simulink model "PIDControllerPulse"  (R2025b)
settings: Solver=FixedStepAuto  StartTime=0.0  StopTime=inf  FixedStep=Ts  RelTol=1e-3
model workspace (MATLAB code in the model file):
  | motor_max_torque = 2.2;
  | gear_ratio = [70/16; 40/16; 1];
  | 
  | u_max =   motor_max_torque * gear_ratio;
  | u_min = - motor_max_torque * gear_ratio;
  | 
  | voltage_max    = 15;
  | torque2voltage = voltage_max ./ u_max;
  | 
  | Ts = 1e-3;
  | pp = 14;
undefined symbols (not defined in the file): effort, effort_SL_Info, position, position_SL_Info
libraries: ros2lib x3, slpidlib x1, eeGeneralControl x1
settings Model: Creator=Asus  LastModifiedBy=Asus
settings OptimizationCC: DefaultParameterBehavior=Inlined  EnhancedBackFolding=on  PassReuseOutputArgsAs=Individual arguments  ZeroExternalMemoryAtStartup=off  ZeroInternalMemoryAtStartup=off  MaxStackSize=64  OptimizeBlockOrder=speed  DifferentSizesBufferReuse=on  OptimizationCustomize=off  EfficientTunableParamExpr=on
settings DebuggingCC: ParameterTunabilityLossMsg=error
settings SFSimCC: MATLABDynamicMemAlloc=off
settings RTWCC: SystemTargetFile=ert.tlc  HardwareBoard=Robot Operating System 2 (ROS 2)  TLCOptions="-aInlineSetEventsForThisBaseRateFcn=TLC_FALSE -aSuppressMultiTaskScheduler=TLC_FALSE  -aRateBasedStepFcn=0"  TemplateMakefile=ert_default_tmf  Toolchain=Colcon Tools  TargetLang=C++  Description=Embedded Coder
settings CodeAppCC: ForceParamTrailComments=on  IgnoreCustomStorageClasses=off  MaxIdLength=95.0  OperatorAnnotations=on  SimulinkDataObjDesc=on  SFDataObjDesc=on  InsertBlockDesc=on
settings ERTTargetCC: RootIOFormat=Structure reference  CodeInterfacePackaging=C++ class

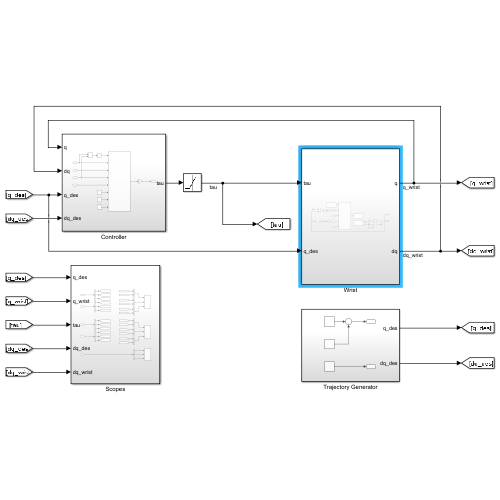
[thumbnail: Simulink's stored preview of the top-level diagram]
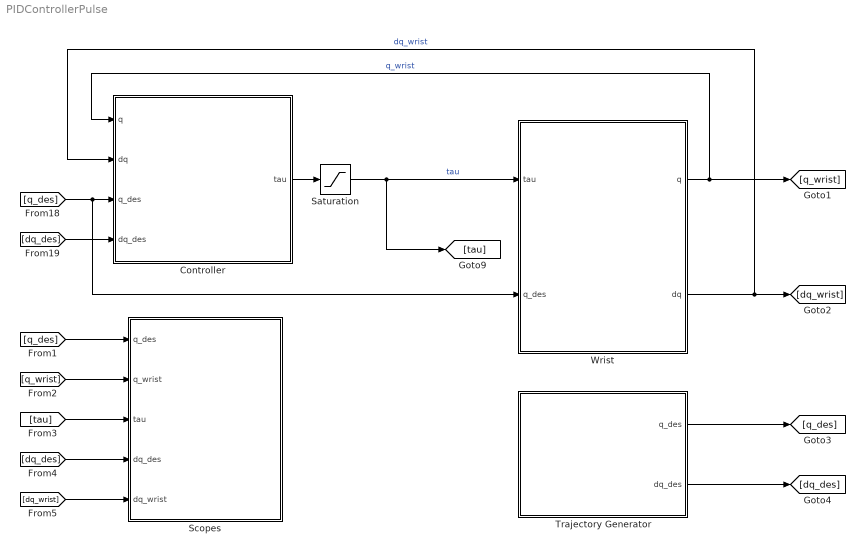
== system PIDControllerPulse ==
  Controller : Subsystem
  Saturation : Saturate  UpperLimit=u_max  LowerLimit=u_min
  Scopes : Subsystem
  Trajectory Generator : Subsystem
  Wrist : Subsystem
  wires:
  [q_des] -> Wrist/2(q_des), Controller/3(q_des)
  [dq_des] -> Controller/4(dq_des)
  Controller/1(tau) -> Saturation/1
  Wrist/1(q) -> Controller/1(q), [q_wrist]  "q_wrist"
  Wrist/2(dq) -> [dq_wrist], Controller/2(dq)  "dq_wrist"
  [q_des] -> Scopes/1(q_des)
  [q_wrist] -> Scopes/2(q_wrist)
  [tau] -> Scopes/3(tau)
  Trajectory Generator/1(q_des) -> [q_des]
  Trajectory Generator/2(dq_des) -> [dq_des]
  [dq_des] -> Scopes/4(dq_des)
  [dq_wrist] -> Scopes/5(dq_wrist)
  Saturation/1 -> [tau], Wrist/1(tau)  "tau"

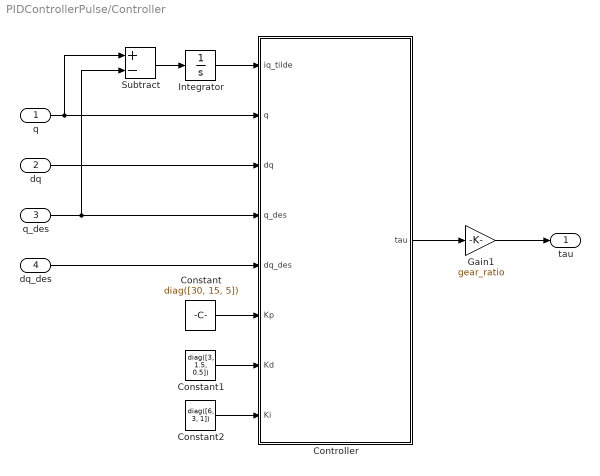
== system PIDControllerPulse/Controller ==
  q : Inport
  dq : Inport  Port=2
  q_des : Inport  Port=3
  dq_des : Inport  Port=4
  Constant : Constant  Value=diag([30, 15, 5])
  Constant1 : Constant  Value=diag([3, 1.5, 0.5])
  Constant2 : Constant  Value=diag([6, 3, 1])
  Controller : MATLAB Function  TreatAsAtomicUnit=on
  Gain1 : Gain  Gain=gear_ratio
  Integrator : Integrator  InitialCondition=zeros(3, 1)
  Subtract : Sum  Inputs=+-
  tau : Outport
  wires:
  q_des/1 -> Subtract/2, Controller/4(q_des)
  dq/1 -> Controller/3(dq)
  q/1 -> Subtract/1, Controller/2(q)
  Constant/1 -> Controller/6(Kp)
  Constant1/1 -> Controller/7(Kd)
  dq_des/1 -> Controller/5(dq_des)
  Subtract/1 -> Integrator/1
  Integrator/1 -> Controller/1(iq_tilde)
  Constant2/1 -> Controller/8(Ki)
  Controller/1(tau) -> Gain1/1
  Gain1/1 -> tau/1

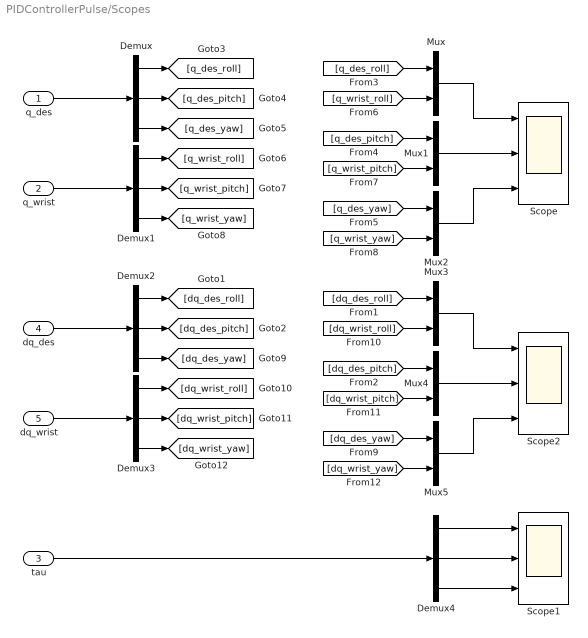
== system PIDControllerPulse/Scopes ==
  q_des : Inport
  q_wrist : Inport  Port=2
  tau : Inport  Port=3
  dq_des : Inport  Port=4
  dq_wrist : Inport  Port=5
  Demux{,1..4} (5 alike) : Demux  Outputs=3
  Mux{,1..5} (6 alike) : Mux  Inputs=2
  Scope : Scope  NumInputPorts=3
      settings: ActiveDisplayYMinimum=-0.31272116573527453  ActiveDisplayYMaximum=0.31449049161747095
  Scope1 : Scope  NumInputPorts=3
      settings: ActiveDisplayYMinimum=-12.03125  ActiveDisplayYMaximum=12.03125
  Scope2 : Scope  NumInputPorts=3
      settings: ActiveDisplayYMinimum=-1  ActiveDisplayYMaximum=1  DataLoggingVariableName=ScopeData2
  wires:
  Demux1/2 -> [q_wrist_pitch]
  q_des/1 -> Demux/1
  Demux/2 -> [q_des_pitch]
  [q_des_roll] -> Mux/1
  Mux1/1 -> Scope/2
  Mux/1 -> Scope/1
  [q_wrist_pitch] -> Mux1/2
  q_wrist/1 -> Demux1/1
  Demux1/1 -> [q_wrist_roll]
  Demux1/3 -> [q_wrist_yaw]
  [q_des_pitch] -> Mux1/1
  [q_des_yaw] -> Mux2/1
  [q_wrist_yaw] -> Mux2/2
  Demux/3 -> [q_des_yaw]
  [q_wrist_roll] -> Mux/2
  Mux2/1 -> Scope/3
  Demux/1 -> [q_des_roll]
  dq_des/1 -> Demux2/1
  dq_wrist/1 -> Demux3/1
  [dq_des_pitch] -> Mux4/1
  Demux2/1 -> [dq_des_roll]
  [dq_wrist_yaw] -> Mux5/2
  [dq_wrist_roll] -> Mux3/2
  [dq_des_yaw] -> Mux5/1
  Mux5/1 -> Scope2/3
  Demux2/3 -> [dq_des_yaw]
  [dq_des_roll] -> Mux3/1
  Demux3/3 -> [dq_wrist_yaw]
  [dq_wrist_pitch] -> Mux4/2
  Demux2/2 -> [dq_des_pitch]
  Mux3/1 -> Scope2/1
  Mux4/1 -> Scope2/2
  Demux3/2 -> [dq_wrist_pitch]
  Demux3/1 -> [dq_wrist_roll]
  tau/1 -> Demux4/1
  Demux4/1 -> Scope1/1
  Demux4/2 -> Scope1/2
  Demux4/3 -> Scope1/3

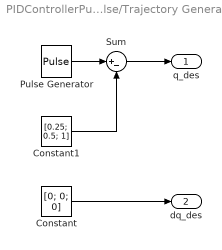
== system PIDControllerPulse/Trajectory Generator ==
  Constant : Constant  Value=[0; 0; 0]
  Constant1 : Constant  Value=[0.25; 0.5; 1]
  Pulse Generator : DiscretePulseGenerator  PulseType=Time based  Amplitude=2 * [0.25; 0.5; 1]  Period=[10; 10; 10]  PulseWidth=50
  Sum : Sum  Inputs=|+-
  q_des : Outport
  dq_des : Outport  Port=2
  wires:
  Constant/1 -> dq_des/1
  Pulse Generator/1 -> Sum/1
  Sum/1 -> q_des/1
  Constant1/1 -> Sum/2

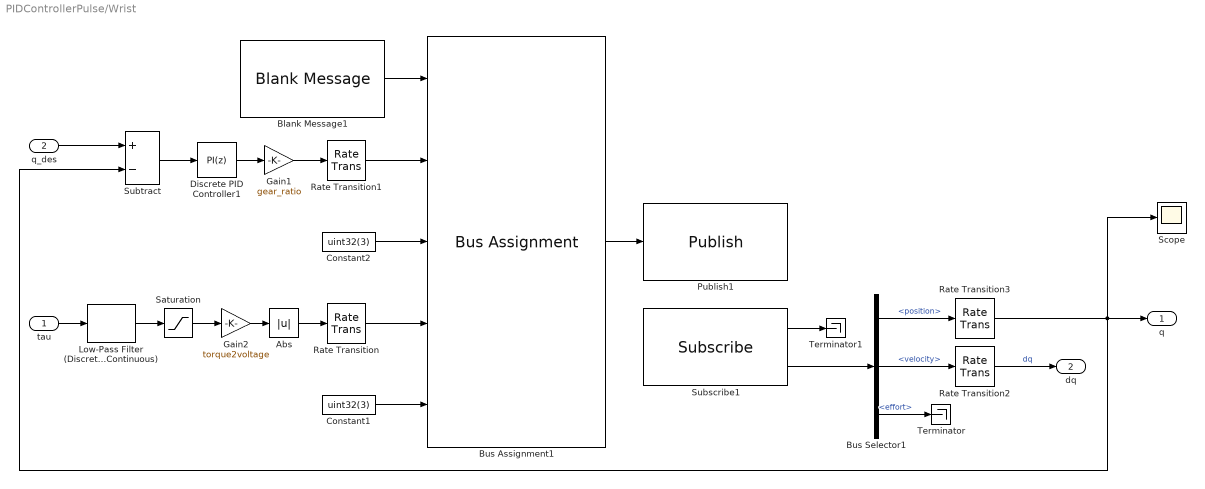
== system PIDControllerPulse/Wrist ==
  tau : Inport
  q_des : Inport  Port=2
  Abs : Abs  SaturateOnIntegerOverflow=off
  Blank Message1 : ros2lib/Blank Message  messageClass=Message  entityType=sensor_msgs/JointState  messageType=sensor_msgs/JointState  SampleTime=0.02
  Bus Assignment1 : BusAssignment  AssignedSignals=position,position_SL_Info.CurrentLength,effort,effort_SL_Info.CurrentLength
  Bus Selector1 : BusSelector  OutputSignals=position,velocity,effort
  Constant1 : Constant  Value=uint32(3)
  Constant2 : Constant  Value=uint32(3)
  Discrete PID Controller1 : slpidlib/PID Controller  Controller=PI  Form=Parallel  TimeDomain=Discrete-time  UseExternalTs=off  SampleTime=-1  IntegratorMethod=Forward Euler  FilterMethod=Forward Euler  ControllerParametersSource=internal  P=0.02  I=20  UseKiTs=off  D=0  UseExternalDerivativeSource=off  N=100  UseFilter=on  TunerSelectOption=Transfer Function Based (PID Tuner App)  InitialConditionSource=internal  InitialConditionForIntegrator=0  InitialConditionForFilter=0  DifferentiatorICPrevScaledInput=0  ExternalReset=none  TrackingMode=off  Kt=1  LimitOutput=off  SatLimitsSource=internal  UpperSaturationLimit=inf  LowerSaturationLimit=-inf  LinearizeAsGain=off  AntiWindupMode=none  Kb=1  LimitIntegrator=off  UpperIntegratorSaturationLimit=inf  LowerIntegratorSaturationLimit=-inf  POutMin=[]  POutMax=[]  IOutMin=[]  IOutMax=[]  DOutMin=[]  DOutMax=[]  NOutMin=[]  NOutMax=[]  SumOutMin=[]  SumOutMax=[]  SaturationOutMin=[]  SaturationOutMax=[]  PParamMin=[]  PParamMax=[]  IParamMin=[]  IParamMax=[]  DParamMin=[]  DParamMax=[]  NParamMin=[]  NParamMax=[]  KbParamMin=[]  KbParamMax=[]  KtParamMin=[]  KtParamMax=[]  KbOutMin=[]  KbOutMax=[]  KtOutMin=[]  KtOutMax=[]  IntegratorOutMin=[]  IntegratorOutMax=[]  FilterOutMin=[]  FilterOutMax=[]  SumI1OutMin=[]  SumI1OutMax=[]  SumI2OutMin=[]  SumI2OutMax=[]  SumI3OutMin=[]  SumI3OutMax=[]  SumI4OutMin=[]  SumI4OutMax=[]  SumDOutMin=[]  SumDOutMax=[]  DifferentiatorOutMin=[]  DifferentiatorOutMax=[]  FilterDiffOutCoefMin=[]  FilterDiffOutCoefMax=[]  ReciprocalOutMin=[]  ReciprocalOutMax=[]  SumDenOutMin=[]  SumDenOutMax=[]  SumNumOutMin=[]  SumNumOutMax=[]  DivideOutMin=[]  DivideOutMax=[]  UdiffTsProdOutMin=[]  UdiffTsProdOutMax=[]  NTsProdOutMin=[]  NTsProdOutMax=[]  UintegralTsProdOutMin=[]  UintegralTsProdOutMax=[]  UngainTsProdOutMin=[]  UngainTsProdOutMax=[]  ClampingZeroOutDataTypeStr=Inherit: Inherit via back propagation  ClampingZeroOutMin=[]  ClampingZeroOutMax=[]  FilterDenConstantOutDataTypeStr=Inherit: Inherit via back propagation  FilterDenConstantOutMin=[]  FilterDenConstantOutMax=[]  PCopyOutDataTypeStr=Inherit: Inherit via back propagation  PCopyOutMin=[]  PCopyOutMax=[]  NCopyOutDataTypeStr=Inherit: Inherit via back propagation  NCopyOutMin=[]  NCopyOutMax=[]  IntegratorContinuousStateAttributes=''  IntegratorStateMustResolveToSignalObject=off  IntegratorRTWStateStorageClass=Auto  FilterContinuousStateAttributes=''  FilterStateMustResolveToSignalObject=off  FilterRTWStateStorageClass=Auto  ParallelPVariant=InternalParameters  IdealPVariant=Disabled  IVariant=InternalParameters  DVariant=Disabled  IntegratorVariant=Discrete  SatVariant=Disabled  AWVariant=Passthrough  PCopyVariant=Disabled  TRVariant=Disabled  FdbkBlocksVariant=Forward  IdealPFdbkVariant=Disabled  SatFdbkVariant=Disabled  DerivativeFilterVariant=Disabled  NVariant=Disabled  NCopyVariant=Disabled_SignalSpec  FilterICVariant=Disabled  IntegratorICVariant=InternalICs  ExternalResetVariant=Disabled  TRSumVariant=Passthrough  SumFdbkVariant=Disabled  SumVariant=Sum_PI  TsampFilterVariant=InternalTs  TsampNgainVariant=Passthrough  TsampIntegralVariant=Disabled_SignalSpec  ExternalSaturationOutDataTypeStr=Inherit: Same as second input  DerivativeSourceVariant=Disabled  PreIntVariant=InternalPreInt
      settings: LibrarySourceBlock=simulink/Discrete/Discrete PID Controller
  Gain1 : Gain  Gain=gear_ratio
  Gain2 : Gain  Gain=torque2voltage
  Low-Pass Filter (Discrete or Continuous) : eeGeneralControl/Low-Pass Filter (Discrete or Continuous)  K=1  T=0.001  B=inf  A=-inf  init_option=Inherited from block input  x0=0  Ts=-1
  Publish1 : ros2lib/Publish  topicSource=Specify your own  topic=/joint_desireds  messageType=sensor_msgs/JointState  QOSHistory=Keep last  QOSDepth=10  QOSReliability=Reliable  QOSDurability=Volatile  QOSDeadline=Inf  QOSLifespan=Inf  QOSLiveliness=Automatic  QOSLeaseDuration=Inf  QOSAvoidROSNamespaceConventions=off
  Rate Transition : RateTransition  OutPortSampleTime=0.02
  Rate Transition1 : RateTransition  OutPortSampleTime=0.02
  Rate Transition2 : RateTransition  OutPortSampleTime=Ts
  Rate Transition3 : RateTransition  OutPortSampleTime=Ts
  Saturation : Saturate  UpperLimit=u_max  LowerLimit=u_min
  Scope : Scope
      settings: ActiveDisplayYMinimum=-1  ActiveDisplayYMaximum=1  DataLoggingVariableName=ScopeData3
  Subscribe1 : ros2lib/Subscribe  topicSource=Select from ROS network  topic=/joint_states  messageType=sensor_msgs/JointState  sampleTime=0.02  QOSHistory=Keep all  QOSDepth=3  QOSReliability=Best effort  QOSDurability=Volatile  QOSDeadline=Inf  QOSLifespan=Inf  QOSLiveliness=Automatic  QOSLeaseDuration=Inf  QOSAvoidROSNamespaceConventions=off
  Subtract : Sum  Inputs=+-
  Terminator : Terminator
  Terminator1 : Terminator
  q : Outport
  dq : Outport  Port=2
  wires:
  Rate Transition1/1 -> Bus Assignment1/2
  Bus Selector1/3 -> Terminator/1  "<effort>"
  Bus Selector1/1 -> Rate Transition3/1  "<position>"
  Rate Transition2/1 -> dq/1  "dq"
  Constant1/1 -> Bus Assignment1/5
  Subscribe1/2 -> Bus Selector1/1
  Rate Transition3/1 -> Scope/1, Subtract/2, q/1
  Blank Message1/1 -> Bus Assignment1/1
  Bus Selector1/2 -> Rate Transition2/1  "<velocity>"
  Constant2/1 -> Bus Assignment1/3
  Abs/1 -> Rate Transition/1
  Subscribe1/1 -> Terminator1/1
  Bus Assignment1/1 -> Publish1/1
  Gain2/1 -> Abs/1
  Rate Transition/1 -> Bus Assignment1/4
  Saturation/1 -> Gain2/1
  Subtract/1 -> Discrete PID Controller1/1
  q_des/1 -> Subtract/1
  Discrete PID Controller1/1 -> Gain1/1
  Gain1/1 -> Rate Transition1/1
  tau/1 -> Low-Pass Filter (Discrete or Continuous)/1
  Low-Pass Filter (Discrete or Continuous)/1 -> Saturation/1

== matlab function PIDControllerPulse/Controller/Controller ==
  data: iq_tilde input; q input; tau output; dq input; q_des input; dq_des input; Kp input; Kd input; Ki input
function tau = fcn(iq_tilde, q, dq, q_des, dq_des, Kp, Kd, Ki)

    q_tilde  = q - q_des;
    dq_tilde = dq - dq_des;
    tau      = - Kp * q_tilde - Kd * dq_tilde - Ki * iq_tilde;

end
